simulink model "D_controller"  (R2018a)
settings: Solver=VariableStepAuto  StartTime=0.0  StopTime=1000  RelTol=1e-3
settings Model: Creator=mjb15180  LastModifiedBy=mjb15180

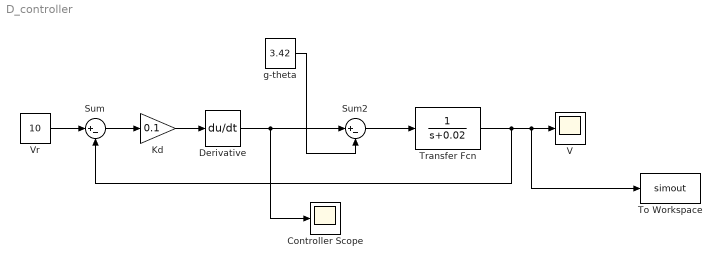
== system D_controller ==
  Controller Scope : Scope
  Derivative : Derivative  CoefficientInTFapproximation=1
  Kd : Gain  Gain=0.1
  Sum : Sum  Inputs=|+-
  Sum2 : Sum  Inputs=|+-
  To Workspace : ToWorkspace  VariableName=simout  SaveFormat=Timeseries  SampleTime=-1
  Transfer Fcn : TransferFcn  Denominator=[1 0.02]
  V : Scope
  Vr : Constant  Value=10
  g-theta : Constant  Value=3.42
  wires:
  Sum2/1 -> Transfer Fcn/1
  Transfer Fcn/1 -> Sum/2, To Workspace/1, V/1
  Derivative/1 -> Sum2/1, Controller Scope/1
  g-theta/1 -> Sum2/2
  Kd/1 -> Derivative/1
  Vr/1 -> Sum/1
  Sum/1 -> Kd/1
